simulink model "DF002A_Swp"  (R2013b)
settings: Solver=FixedStepDiscrete  StartTime=0  StopTime=350  FixedStep=ARCHGLBPRM_2MILLISEC_SEC_F32  RelTol=1e-3
undefined symbols (not defined in the file): ARCHGLBPRM_2MILLISEC_SEC_F32, ARCHGLBPRM_2PI_ULS_F32, SwpCfg, SwpDwellTi, SwpFrqList, SwpGain, SwpModEna, SwpOffs, SwpSinAmp, SWPTIUNITCNVN, SwpTranTi, SwpVehSpdChkEna, SwpVehSpdMax
libraries: simulink x6, NexteerUtilities x2
(part 2 of 2)

== system DF002A_Swp/Swp/DF002A Sweep Function/ SwpPer1/Check GenHwTrq and VehSpd/If GenHwTrq=TRUE, Check Vehicle Speed Criteria/Switch Case Block/Dwell//Stop: Switch Case Action Subsystem1/Cosine Calculation ==
  note: This constant defined as a
      | PIM in data dictionary
  note: This constant defined as a
      | PIM in data dictionary
  SinArg : Inport
  SF : Inport  Port=2
  Constant1 : Constant  Value=SwpSinAmp
  Constant3 : Constant  Value=SwpOffs
  Gain2 : Gain  Gain=ARCHGLBPRM_2PI_ULS_F32
  Product1 : Product  RndMeth=Zero
  Product2 : Product  RndMeth=Zero
  Sum4 : Sum  Inputs=|++
  Trigonometric Function : Trigonometry  Operator=cos
  Out1 : Outport
  wires:
  Gain2/1 -> Trigonometric Function/1
  Product2/1 -> Out1/1
  SinArg/1 -> Gain2/1
  Sum4/1 -> Product2/1
  Product1/1 -> Sum4/1
  Trigonometric Function/1 -> Product1/2
  SF/1 -> Product2/2
  Constant1/1 -> Product1/1  "SwpSinAmp"
  Constant3/1 -> Sum4/2  "SwpOffs"

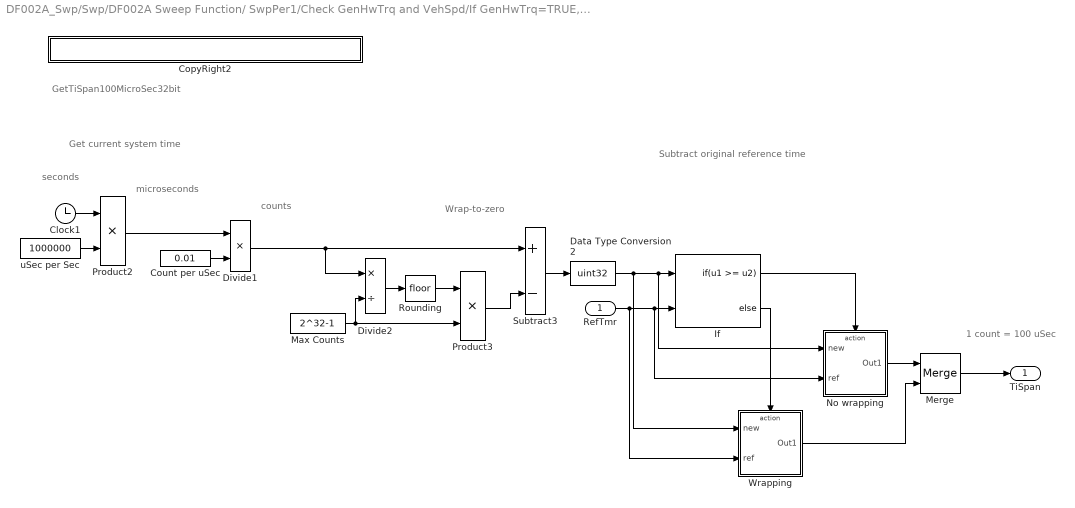
== system DF002A_Swp/Swp/DF002A Sweep Function/ SwpPer1/Check GenHwTrq and VehSpd/If GenHwTrq=TRUE, Check Vehicle Speed Criteria/Switch Case Block/Dwell//Stop: Switch Case Action Subsystem1/GetTiSpan100MicroSec32bit1 ==
  note: GetTiSpan100MicroSec32bit
  note: Get current system time
  note: 1 count = 100 uSec
  note: Wrap-to-zero
  note: counts
  note: microseconds
  note: seconds
  note: Subtract original reference time
  RefTmr : Inport
  Clock1 : Clock
  CopyRight2 : Subsystem  Description=|  mask(Copyright Information){none=on}
      | Copyright info block.                                               
      |                                                                     
      | Place copyright information at the top of every subsystem in design.
      mask prompts: none "No parameters"
      mask help: Place copyright information at the top of every subsystem in design.
      mask Display:
      | NxtrConf = 'Nexteer Confidential';
      | 
      | sys = bdroot; %handle for the current model ("system")
      | first = get_param(sys,'Created');
      | if(isempty(first))
      |     first = datestr(now,'yyyy');
      | else
      |     first = first(end-3:end);  %year is last four digits
      | end
      | 
      | last = get_param(sys,'LastModifiedDate');
      | if isempty(last)
      |     last = datestr(now,'yyyy');
      | else
      |     last = last(end-3:end);
      | end
      | 
      | if strcmp(first,last)
      |     fprintf('%s -- Copyright %s Nexteer',NxtrConf,first)
      | else
      |     fprintf('%s -- %s%s- %s Nexteer',NxtrConf,char(169),first,last)
      | end
  Count per uSec : Constant  Value=0.01
  Data Type Conversion2 : DataTypeConversion  OutDataTypeStr=uint32
  Divide1 : Product  Inputs=**
  Divide2 : Product  Inputs=*/
  If : If  NumInputs=2  IfExpression=u1 >= u2
  Max Counts : Constant  Value=2^32-1
  Merge : Merge
  No wrapping : Subsystem  TreatAsAtomicUnit=on
  Product2 : Product
  Product3 : Product
  Rounding : Rounding
  Subtract3 : Sum  Inputs=+-
  Wrapping : Subsystem  TreatAsAtomicUnit=on
  uSec per Sec : Constant  Value=1000000
  TiSpan : Outport
  wires:
  Data Type Conversion2/1 -> Wrapping/1(new), No wrapping/1(new), If/1
  RefTmr/1 -> Wrapping/2(ref), No wrapping/2(ref), If/2
  Merge/1 -> TiSpan/1
  uSec per Sec/1 -> Product2/2
  Count per uSec/1 -> Divide1/2
  Clock1/1 -> Product2/1
  Product2/1 -> Divide1/1
  Divide1/1 -> Subtract3/1, Divide2/1
  Max Counts/1 -> Product3/2, Divide2/2
  Divide2/1 -> Rounding/1
  Rounding/1 -> Product3/1
  Subtract3/1 -> Data Type Conversion2/1
  Product3/1 -> Subtract3/2
  If/1 -> No wrapping/Action
  If/2 -> Wrapping/Action
  No wrapping/1(Out1) -> Merge/1
  Wrapping/1(Out1) -> Merge/2

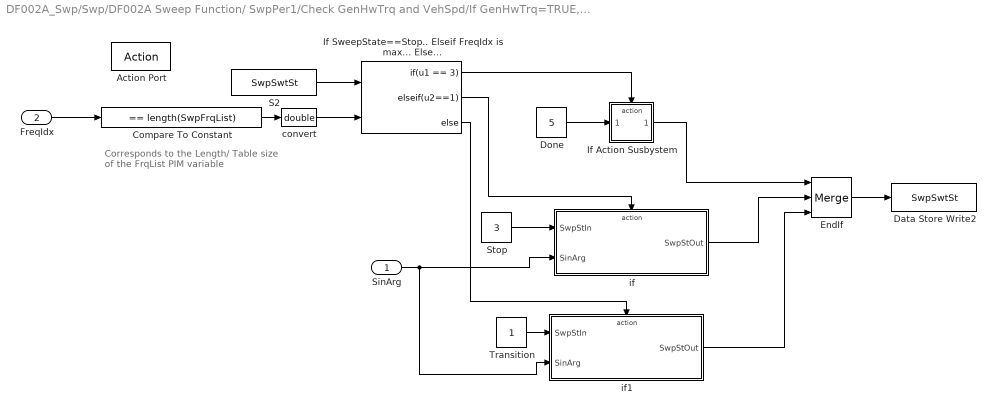
== system DF002A_Swp/Swp/DF002A Sweep Function/ SwpPer1/Check GenHwTrq and VehSpd/If GenHwTrq=TRUE, Check Vehicle Speed Criteria/Switch Case Block/Dwell//Stop: Switch Case Action Subsystem1/If Action Subsystem ==
  note: Corresponds to the Length/ Table size
      | of the FrqList  PIM variable
  SinArg : Inport
  FreqIdx : Inport  Port=2
  Action Port : ActionPort  ActionType=then
  Compare To Constant : simulink/Logic and Bit Operations/Compare To Constant  relop===  const=length(SwpFrqList)  OutDataTypeStr=boolean
      settings: AttributesFormatString=%<const>
  Data Store Write2 : DataStoreWrite  RequirementInfo={} %GIDa_98c06136_1203_45eb_bd39_84f10c760bb6  DataStoreName=SwpSwtSt
  Done : Constant  Value=5
  EndIf : Merge  Inputs=3
  If Action Susbystem : Subsystem  TreatAsAtomicUnit=on  mask(pass thru, version Nov 30, 2012){nIn=1}
      mask prompts: nIn "Number of input signals"
      mask help:
      | This block passes its input straight through without modification.
      |
      | Enter the number of signals to pass through (integer 1 to 5).
      mask Callback nIn:
      | thisBlock = gcb;
      | a = get_param(thisBlock,'MaskValues');
      | b = cell2mat(a);
      | c = str2num(b);
      | 
      | if c<1 c=1; end
      | if c>5 c=5; end
      | 
      | for idx=1:c
      |     sIdx = num2str(idx);
      |     oldblock = [thisBlock '/In' sIdx];
      |     if strcmp(get_param(oldblock,'BlockType'),'Ground')
      |          newblock = 'built-in/Inport';
      |         pos = get_param(oldblock,'Position');
      |         orient = get_param(oldblock,'Orientation');
      |         delete_block(oldblock);
      |         add_block(newblock,oldblock,'Position',pos, 'Orientation',orient);
      |     end
      | 
      |     oldblock = [thisBlock '/Out' sIdx];
      |     if strcmp(get_param(oldblock,'BlockType'),'Terminator')
      |         newblock = 'built-in/Outport';
      |         pos = get_param(oldblock,'Position');
      |         orient = get_param(oldblock,'Orientation');
      |         delete_block(oldblock);
      |         add_block(newblock,oldblock,'Position',pos, 'Orientation',orient);
      |     end
      | end
      | 
      | for idx=c+1:5
      |     sIdx = num2str(idx);
      |     oldblock = [thisBlock '/In' sIdx];
      |     if strcmp(get_param(oldblock,'BlockType'),'Inport')
      |         newblock = 'built-in/Ground';
      |         pos = get_param(oldblock,'Position');
      |         orient = get_param(oldblock,'Orientation');
      |         delete_block(oldblock);
      |         add_block(newblock,oldblock,'Position',pos, 'Orientation',orient);
      |     end
      | 
      |     oldblock = [thisBlock '/Out' sIdx];
      |     if strcmp(get_param(oldblock,'BlockType'),'Outport')
      |         newblock = 'built-in/Terminator';
      |         pos = get_param(oldblock,'Position');
      |         orient = get_param(oldblock,'Orientation');
      |         delete_block(oldblock);
      |         add_block(newblock,oldblock,'Position',pos, 'Orientation',orient);
      |     end
      | end
      | 
      | 
      | 
      | clear thisBlock oldblock newblock orient pos a b c idx sIdx ;
      mask Display: fprintf('pass\nthru')
  If SweepState==Stop.. Elseif FreqIdx is max... Else... : If  NumInputs=2  IfExpression=u1 == 3  ElseIfExpressions=u2==1
  S2 : DataStoreRead  DataStoreName=SwpSwtSt
  Stop : Constant  Value=3
  Transition : Constant
  convert : DataTypeConversion  OutDataTypeStr=double
  if : Subsystem  RequirementInfo={} %GIDa_0dc71279_9bfd_4c7e_903f_84cae79553a4  TreatAsAtomicUnit=on
  if1 : Subsystem  RequirementInfo={} %GIDa_9f322384_3993_4c4c_ad2a_ea70a5303c05  TreatAsAtomicUnit=on
  wires:
  S2/1 -> If SweepState==Stop.. Elseif FreqIdx is max... Else.../1
  If Action Susbystem/1(Out1) -> EndIf/1
  EndIf/1 -> Data Store Write2/1
  Done/1 -> If Action Susbystem/1(In1)
  If SweepState==Stop.. Elseif FreqIdx is max... Else.../1 -> If Action Susbystem/Action
  If SweepState==Stop.. Elseif FreqIdx is max... Else.../2 -> if/Action
  If SweepState==Stop.. Elseif FreqIdx is max... Else.../3 -> if1/Action
  FreqIdx/1 -> Compare To Constant/1
  Compare To Constant/1 -> convert/1
  convert/1 -> If SweepState==Stop.. Elseif FreqIdx is max... Else.../2
  Stop/1 -> if/1(SwpStIn)
  Transition/1 -> if1/1(SwpStIn)
  if/1(SwpStOut) -> EndIf/2
  if1/1(SwpStOut) -> EndIf/3
  SinArg/1 -> if1/2(SinArg), if/2(SinArg)

== system DF002A_Swp/Swp/DF002A Sweep Function/ SwpPer1/Check GenHwTrq and VehSpd/If GenHwTrq=TRUE, Check Vehicle Speed Criteria/Switch Case Block/Dwell//Stop: Switch Case Action Subsystem1/If Action Subsystem1 ==
  TransitionTime : Inport
  TimeScale : Inport  Port=2
  Action Port : ActionPort  ActionType=then
  Constant1 : Constant
  Sum : Sum  Inputs=|-+
  ScaleFactor : Outport
  StateTime : Outport  Port=2
  wires:
  TimeScale/1 -> Sum/1  "TimeScale_Uls_T_f32"
  Constant1/1 -> Sum/2
  TransitionTime/1 -> StateTime/1
  Sum/1 -> ScaleFactor/1

== system DF002A_Swp/Swp/DF002A Sweep Function/ SwpPer1/Check GenHwTrq and VehSpd/If GenHwTrq=TRUE, Check Vehicle Speed Criteria/Switch Case Block/Dwell//Stop: Switch Case Action Subsystem1/If Action Subsystem2 ==
  DwellTime : Inport
  Action Port : ActionPort  ActionType=else
  Constant2 : Constant
  ScaleFactor : Outport
  StateTime : Outport  Port=2
  wires:
  DwellTime/1 -> StateTime/1
  Constant2/1 -> ScaleFactor/1

== system DF002A_Swp/Swp/DF002A Sweep Function/ SwpPer1/Check GenHwTrq and VehSpd/If GenHwTrq=TRUE, Check Vehicle Speed Criteria/Switch Case Block/Dwell//Stop: Switch Case Action Subsystem1/Inst Frequency Calculation ==
  note: This block find instantaneous frequency of the sinusoid signal during dwell/stop case.
      | Since the frequency is held constand during either of these cases, InstFreq=CurrentFreq
  CurrentFreq : Inport
  InstFreq : Outport
  wires:
  CurrentFreq/1 -> InstFreq/1

== system DF002A_Swp/Swp/DF002A Sweep Function/ SwpPer1/Check GenHwTrq and VehSpd/If GenHwTrq=TRUE, Check Vehicle Speed Criteria/Switch Case Block/Dwell//Stop: Switch Case Action Subsystem1/Sine Calculation ==
  note: This constant defined as a
      | PIM in data dictionary
  note: This constant defined as a
      | PIM in data dictionary
  SinArg : Inport
  SF : Inport  Port=2
  Constant3 : Constant  Value=SwpOffs
  Constant4 : Constant  Value=SwpSinAmp
  Gain2 : Gain  Gain=ARCHGLBPRM_2PI_ULS_F32
  Product1 : Product  RndMeth=Zero
  Product2 : Product  RndMeth=Zero
  Sum4 : Sum  Inputs=|++
  Trigonometric Function : Trigonometry
  Out1 : Outport
  wires:
  Gain2/1 -> Trigonometric Function/1
  Product2/1 -> Out1/1
  SinArg/1 -> Gain2/1
  Sum4/1 -> Product2/1
  Product1/1 -> Sum4/1
  Constant4/1 -> Product1/1  "SwpSinAmp"
  Trigonometric Function/1 -> Product1/2
  SF/1 -> Product2/2
  Constant3/1 -> Sum4/2  "SwpOffs"

== system DF002A_Swp/Swp/DF002A Sweep Function/ SwpPer1/Check GenHwTrq and VehSpd/If GenHwTrq=TRUE, Check Vehicle Speed Criteria/Switch Case Block/Ramp: Switch Case Action/Else Action Subsystem ==
  SweepTorqueIn : Inport
  CosSweepTorqueIn : Inport  Port=2
  ScaleFactor : Inport  Port=3
  Action Port : ActionPort  ActionType=else
  Product : Product  RndMeth=Zero
  Product1 : Product  RndMeth=Zero
  SweepTorque : Outport
  CosSweepTorque : Outport  Port=2
  wires:
  CosSweepTorqueIn/1 -> Product1/2
  ScaleFactor/1 -> Product/2, Product1/1
  Product/1 -> SweepTorque/1
  Product1/1 -> CosSweepTorque/1
  SweepTorqueIn/1 -> Product/1

== system DF002A_Swp/Swp/DF002A Sweep Function/ SwpPer1/Check GenHwTrq and VehSpd/If GenHwTrq=TRUE, Check Vehicle Speed Criteria/Switch Case Block/Ramp: Switch Case Action/Else Action Subsystem1 ==
  Action Port : ActionPort  ActionType=then
  Constant : Constant  Value=0
  Constant1 : Constant  Value=0
  Data Store Write2 : DataStoreWrite  RequirementInfo={} %GIDa_95120470_507b_4450_bc77_8b8934b75d51  DataStoreName=SwpSwtSt
  DefaultSweepState (DONE) : Constant  Value=5
  SweepTorque : Outport
  CosSweepTorque : Outport  Port=2
  wires:
  Constant/1 -> SweepTorque/1
  Constant1/1 -> CosSweepTorque/1
  DefaultSweepState (DONE)/1 -> Data Store Write2/1

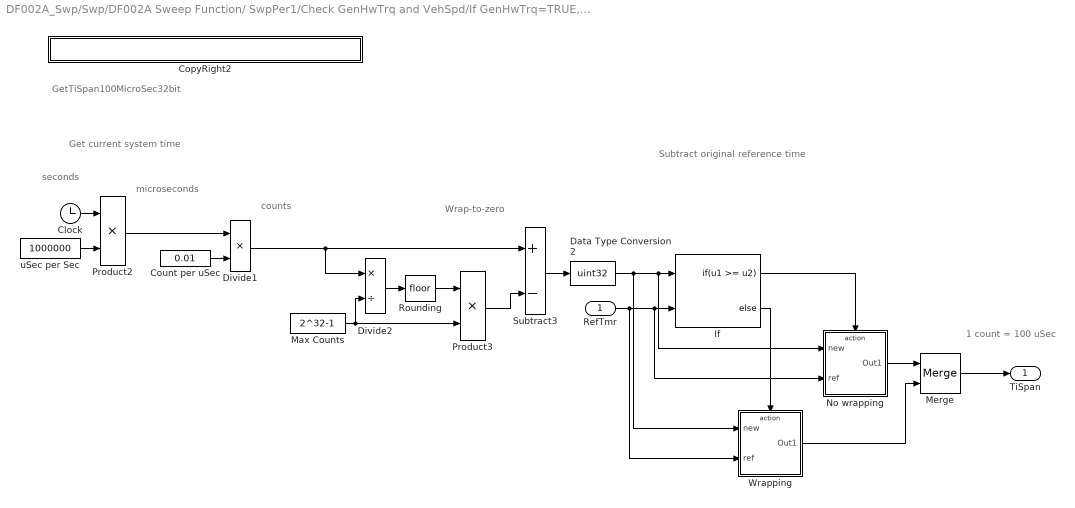
== system DF002A_Swp/Swp/DF002A Sweep Function/ SwpPer1/Check GenHwTrq and VehSpd/If GenHwTrq=TRUE, Check Vehicle Speed Criteria/Switch Case Block/Ramp: Switch Case Action/GetTiSpan100MicroSec32bit1 ==
  note: GetTiSpan100MicroSec32bit
  note: Get current system time
  note: 1 count = 100 uSec
  note: Wrap-to-zero
  note: counts
  note: microseconds
  note: seconds
  note: Subtract original reference time
  RefTmr : Inport
  Clock : Clock
  CopyRight2 : Subsystem  Description=|  mask(Copyright Information){none=on}
      | Copyright info block.                                               
      |                                                                     
      | Place copyright information at the top of every subsystem in design.
      mask prompts: none "No parameters"
      mask help: Place copyright information at the top of every subsystem in design.
      mask Display:
      | NxtrConf = 'Nexteer Confidential';
      | 
      | sys = bdroot; %handle for the current model ("system")
      | first = get_param(sys,'Created');
      | if(isempty(first))
      |     first = datestr(now,'yyyy');
      | else
      |     first = first(end-3:end);  %year is last four digits
      | end
      | 
      | last = get_param(sys,'LastModifiedDate');
      | if isempty(last)
      |     last = datestr(now,'yyyy');
      | else
      |     last = last(end-3:end);
      | end
      | 
      | if strcmp(first,last)
      |     fprintf('%s -- Copyright %s Nexteer',NxtrConf,first)
      | else
      |     fprintf('%s -- %s%s- %s Nexteer',NxtrConf,char(169),first,last)
      | end
  Count per uSec : Constant  Value=0.01
  Data Type Conversion2 : DataTypeConversion  OutDataTypeStr=uint32
  Divide1 : Product  Inputs=**
  Divide2 : Product  Inputs=*/
  If : If  NumInputs=2  IfExpression=u1 >= u2
  Max Counts : Constant  Value=2^32-1
  Merge : Merge
  No wrapping : Subsystem  TreatAsAtomicUnit=on
  Product2 : Product
  Product3 : Product
  Rounding : Rounding
  Subtract3 : Sum  Inputs=+-
  Wrapping : Subsystem  TreatAsAtomicUnit=on
  uSec per Sec : Constant  Value=1000000
  TiSpan : Outport
  wires:
  Data Type Conversion2/1 -> Wrapping/1(new), No wrapping/1(new), If/1
  RefTmr/1 -> Wrapping/2(ref), No wrapping/2(ref), If/2
  Merge/1 -> TiSpan/1
  uSec per Sec/1 -> Product2/2
  Count per uSec/1 -> Divide1/2
  Clock/1 -> Product2/1
  Product2/1 -> Divide1/1
  Divide1/1 -> Subtract3/1, Divide2/1
  Max Counts/1 -> Product3/2, Divide2/2
  Divide2/1 -> Rounding/1
  Rounding/1 -> Product3/1
  Subtract3/1 -> Data Type Conversion2/1
  Product3/1 -> Subtract3/2
  If/1 -> No wrapping/Action
  If/2 -> Wrapping/Action
  No wrapping/1(Out1) -> Merge/1
  Wrapping/1(Out1) -> Merge/2

== system DF002A_Swp/Swp/DF002A Sweep Function/ SwpPer1/Check GenHwTrq and VehSpd/If GenHwTrq=TRUE, Check Vehicle Speed Criteria/Switch Case Block/Start//Transition: Switch Case Action Subsystem /Cosine Calculation ==
  note: This constant defined as a
      | PIM in data dictionary
  note: This constant defined as a
      | PIM in data dictionary
  SF : Inport
  SinArg : Inport  Port=2
  Constant3 : Constant  Value=SwpOffs
  Constant4 : Constant  Value=SwpSinAmp
  Gain2 : Gain  Gain=ARCHGLBPRM_2PI_ULS_F32
  Product1 : Product  RndMeth=Zero
  Product2 : Product  RndMeth=Zero
  Sum4 : Sum  Inputs=|++
  Trigonometric Function : Trigonometry  Operator=cos
  Out1 : Outport
  wires:
  Gain2/1 -> Trigonometric Function/1
  Product2/1 -> Out1/1
  SinArg/1 -> Gain2/1
  Sum4/1 -> Product2/1
  Product1/1 -> Sum4/1
  Trigonometric Function/1 -> Product1/2
  Constant3/1 -> Sum4/2  "SwpOffs"
  SF/1 -> Product2/2
  Constant4/1 -> Product1/1  "SwpSinAmp"

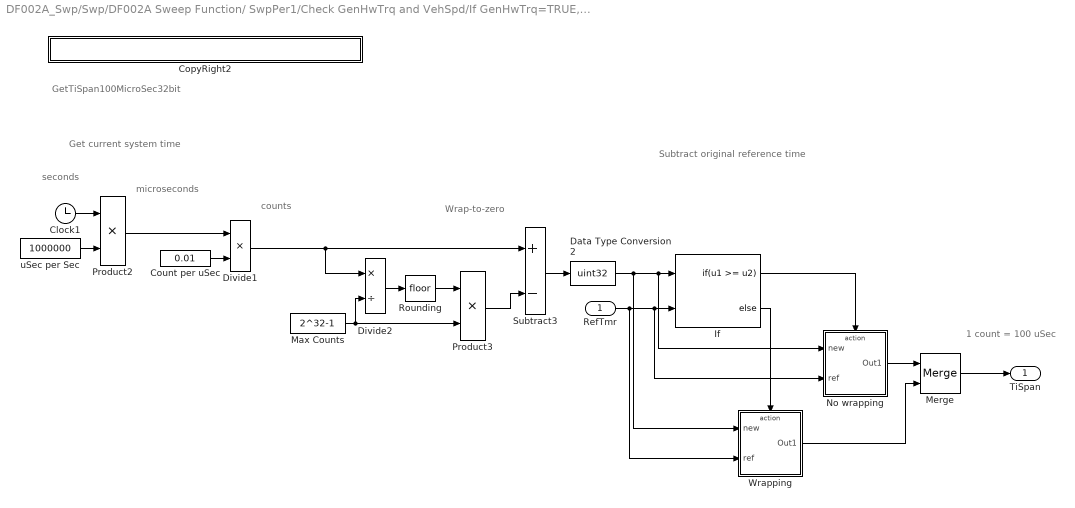
== system DF002A_Swp/Swp/DF002A Sweep Function/ SwpPer1/Check GenHwTrq and VehSpd/If GenHwTrq=TRUE, Check Vehicle Speed Criteria/Switch Case Block/Start//Transition: Switch Case Action Subsystem /GetTiSpan100MicroSec32bit1 ==
  note: GetTiSpan100MicroSec32bit
  note: Get current system time
  note: 1 count = 100 uSec
  note: Wrap-to-zero
  note: counts
  note: microseconds
  note: seconds
  note: Subtract original reference time
  RefTmr : Inport
  Clock1 : Clock
  CopyRight2 : Subsystem  Description=|  mask(Copyright Information){none=on}
      | Copyright info block.                                               
      |                                                                     
      | Place copyright information at the top of every subsystem in design.
      mask prompts: none "No parameters"
      mask help: Place copyright information at the top of every subsystem in design.
      mask Display:
      | NxtrConf = 'Nexteer Confidential';
      | 
      | sys = bdroot; %handle for the current model ("system")
      | first = get_param(sys,'Created');
      | if(isempty(first))
      |     first = datestr(now,'yyyy');
      | else
      |     first = first(end-3:end);  %year is last four digits
      | end
      | 
      | last = get_param(sys,'LastModifiedDate');
      | if isempty(last)
      |     last = datestr(now,'yyyy');
      | else
      |     last = last(end-3:end);
      | end
      | 
      | if strcmp(first,last)
      |     fprintf('%s -- Copyright %s Nexteer',NxtrConf,first)
      | else
      |     fprintf('%s -- %s%s- %s Nexteer',NxtrConf,char(169),first,last)
      | end
  Count per uSec : Constant  Value=0.01
  Data Type Conversion2 : DataTypeConversion  OutDataTypeStr=uint32
  Divide1 : Product  Inputs=**
  Divide2 : Product  Inputs=*/
  If : If  NumInputs=2  IfExpression=u1 >= u2
  Max Counts : Constant  Value=2^32-1
  Merge : Merge
  No wrapping : Subsystem  TreatAsAtomicUnit=on
  Product2 : Product
  Product3 : Product
  Rounding : Rounding
  Subtract3 : Sum  Inputs=+-
  Wrapping : Subsystem  TreatAsAtomicUnit=on
  uSec per Sec : Constant  Value=1000000
  TiSpan : Outport
  wires:
  Data Type Conversion2/1 -> Wrapping/1(new), No wrapping/1(new), If/1
  RefTmr/1 -> Wrapping/2(ref), No wrapping/2(ref), If/2
  Merge/1 -> TiSpan/1
  uSec per Sec/1 -> Product2/2
  Count per uSec/1 -> Divide1/2
  Clock1/1 -> Product2/1
  Product2/1 -> Divide1/1
  Divide1/1 -> Subtract3/1, Divide2/1
  Max Counts/1 -> Product3/2, Divide2/2
  Divide2/1 -> Rounding/1
  Rounding/1 -> Product3/1
  Subtract3/1 -> Data Type Conversion2/1
  Product3/1 -> Subtract3/2
  If/1 -> No wrapping/Action
  If/2 -> Wrapping/Action
  No wrapping/1(Out1) -> Merge/1
  Wrapping/1(Out1) -> Merge/2

== system DF002A_Swp/Swp/DF002A Sweep Function/ SwpPer1/Check GenHwTrq and VehSpd/If GenHwTrq=TRUE, Check Vehicle Speed Criteria/Switch Case Block/Start//Transition: Switch Case Action Subsystem /Inst Frequency Calculation ==
  note: This block find instantaneous frequency of the sinusoid signal during start/transition case.
  TimeScale : Inport
  InitialFreq : Inport  Port=2
  FreqSpan : Inport  Port=3
  Product1 : Product  RndMeth=Zero
  Sum4 : Sum
  InstFreq : Outport
  wires:
  FreqSpan/1 -> Product1/1
  Sum4/1 -> InstFreq/1
  TimeScale/1 -> Product1/2
  Product1/1 -> Sum4/1  "DeltaFreq"
  InitialFreq/1 -> Sum4/2

== system DF002A_Swp/Swp/DF002A Sweep Function/ SwpPer1/Check GenHwTrq and VehSpd/If GenHwTrq=TRUE, Check Vehicle Speed Criteria/Switch Case Block/Start//Transition: Switch Case Action Subsystem /ScaleFactor Calculation ==
  note: Note: FreqIdx starts with 1 in MATLAB. For C code one may have to use 0 as starting index.
  TimeScale : Inport
  FreqIdx : Inport  Port=2
  Constant1 : Constant
  If : If  IfExpression=u1 == 1
  If Action Subsystem : Subsystem  TreatAsAtomicUnit=on  mask(pass thru, version Nov 30, 2012){nIn=1}
      mask prompts: nIn "Number of input signals"
      mask help:
      | This block passes its input straight through without modification.
      |
      | Enter the number of signals to pass through (integer 1 to 5).
      mask Callback nIn:
      | thisBlock = gcb;
      | a = get_param(thisBlock,'MaskValues');
      | b = cell2mat(a);
      | c = str2num(b);
      | 
      | if c<1 c=1; end
      | if c>5 c=5; end
      | 
      | for idx=1:c
      |     sIdx = num2str(idx);
      |     oldblock = [thisBlock '/In' sIdx];
      |     if strcmp(get_param(oldblock,'BlockType'),'Ground')
      |          newblock = 'built-in/Inport';
      |         pos = get_param(oldblock,'Position');
      |         orient = get_param(oldblock,'Orientation');
      |         delete_block(oldblock);
      |         add_block(newblock,oldblock,'Position',pos, 'Orientation',orient);
      |     end
      | 
      |     oldblock = [thisBlock '/Out' sIdx];
      |     if strcmp(get_param(oldblock,'BlockType'),'Terminator')
      |         newblock = 'built-in/Outport';
      |         pos = get_param(oldblock,'Position');
      |         orient = get_param(oldblock,'Orientation');
      |         delete_block(oldblock);
      |         add_block(newblock,oldblock,'Position',pos, 'Orientation',orient);
      |     end
      | end
      | 
      | for idx=c+1:5
      |     sIdx = num2str(idx);
      |     oldblock = [thisBlock '/In' sIdx];
      |     if strcmp(get_param(oldblock,'BlockType'),'Inport')
      |         newblock = 'built-in/Ground';
      |         pos = get_param(oldblock,'Position');
      |         orient = get_param(oldblock,'Orientation');
      |         delete_block(oldblock);
      |         add_block(newblock,oldblock,'Position',pos, 'Orientation',orient);
      |     end
      | 
      |     oldblock = [thisBlock '/Out' sIdx];
      |     if strcmp(get_param(oldblock,'BlockType'),'Outport')
      |         newblock = 'built-in/Terminator';
      |         pos = get_param(oldblock,'Position');
      |         orient = get_param(oldblock,'Orientation');
      |         delete_block(oldblock);
      |         add_block(newblock,oldblock,'Position',pos, 'Orientation',orient);
      |     end
      | end
      | 
      | 
      | 
      | clear thisBlock oldblock newblock orient pos a b c idx sIdx ;
      mask Display: fprintf('pass\nthru')
  ScaleFactorMerge : Merge
  Then Action Subsystem : Subsystem  TreatAsAtomicUnit=on  mask(pass thru, version Nov 30, 2012){nIn=1}
      mask prompts: nIn "Number of input signals"
      mask help:
      | This block passes its input straight through without modification.
      |
      | Enter the number of signals to pass through (integer 1 to 5).
      mask Callback nIn:
      | thisBlock = gcb;
      | a = get_param(thisBlock,'MaskValues');
      | b = cell2mat(a);
      | c = str2num(b);
      | 
      | if c<1 c=1; end
      | if c>5 c=5; end
      | 
      | for idx=1:c
      |     sIdx = num2str(idx);
      |     oldblock = [thisBlock '/In' sIdx];
      |     if strcmp(get_param(oldblock,'BlockType'),'Ground')
      |          newblock = 'built-in/Inport';
      |         pos = get_param(oldblock,'Position');
      |         orient = get_param(oldblock,'Orientation');
      |         delete_block(oldblock);
      |         add_block(newblock,oldblock,'Position',pos, 'Orientation',orient);
      |     end
      | 
      |     oldblock = [thisBlock '/Out' sIdx];
      |     if strcmp(get_param(oldblock,'BlockType'),'Terminator')
      |         newblock = 'built-in/Outport';
      |         pos = get_param(oldblock,'Position');
      |         orient = get_param(oldblock,'Orientation');
      |         delete_block(oldblock);
      |         add_block(newblock,oldblock,'Position',pos, 'Orientation',orient);
      |     end
      | end
      | 
      | for idx=c+1:5
      |     sIdx = num2str(idx);
      |     oldblock = [thisBlock '/In' sIdx];
      |     if strcmp(get_param(oldblock,'BlockType'),'Inport')
      |         newblock = 'built-in/Ground';
      |         pos = get_param(oldblock,'Position');
      |         orient = get_param(oldblock,'Orientation');
      |         delete_block(oldblock);
      |         add_block(newblock,oldblock,'Position',pos, 'Orientation',orient);
      |     end
      | 
      |     oldblock = [thisBlock '/Out' sIdx];
      |     if strcmp(get_param(oldblock,'BlockType'),'Outport')
      |         newblock = 'built-in/Terminator';
      |         pos = get_param(oldblock,'Position');
      |         orient = get_param(oldblock,'Orientation');
      |         delete_block(oldblock);
      |         add_block(newblock,oldblock,'Position',pos, 'Orientation',orient);
      |     end
      | end
      | 
      | 
      | 
      | clear thisBlock oldblock newblock orient pos a b c idx sIdx ;
      mask Display: fprintf('pass\nthru')
  ScaleFactor : Outport
  wires:
  If/2 -> Then Action Subsystem/Action
  Constant1/1 -> Then Action Subsystem/1(In1)
  If Action Subsystem/1(Out1) -> ScaleFactorMerge/1
  Then Action Subsystem/1(Out1) -> ScaleFactorMerge/2
  TimeScale/1 -> If Action Subsystem/1(In1)
  FreqIdx/1 -> If/1
  ScaleFactorMerge/1 -> ScaleFactor/1
  If/1 -> If Action Subsystem/Action

== system DF002A_Swp/Swp/DF002A Sweep Function/ SwpPer1/Check GenHwTrq and VehSpd/If GenHwTrq=TRUE, Check Vehicle Speed Criteria/Switch Case Block/Start//Transition: Switch Case Action Subsystem /Sine Calculation ==
  note: This constant defined as a
      | PIM in data dictionary
  note: This constant defined as a
      | PIM in data dictionary
  SinArg : Inport
  SF : Inport  Port=2
  Constant3 : Constant  Value=SwpOffs
  Constant4 : Constant  Value=SwpSinAmp
  Gain2 : Gain  Gain=ARCHGLBPRM_2PI_ULS_F32
  Product1 : Product  RndMeth=Zero
  Product2 : Product  RndMeth=Zero
  Sum4 : Sum
  Trigonometric Function : Trigonometry
  Out1 : Outport
  wires:
  Gain2/1 -> Trigonometric Function/1
  Product2/1 -> Out1/1
  SinArg/1 -> Gain2/1
  Sum4/1 -> Product2/1
  Product1/1 -> Sum4/1
  Trigonometric Function/1 -> Product1/2
  SF/1 -> Product2/2
  Constant4/1 -> Product1/1  "SwpSinAmp"
  Constant3/1 -> Sum4/2  "SwpOffs"

== system DF002A_Swp/Swp/DF002A Sweep Function/ SwpPer1/Check GenHwTrq and VehSpd/If GenHwTrq=TRUE, Check Vehicle Speed Criteria/Switch Case Block/Start//Transition: Switch Case Action Subsystem /if ==
  SwpStIn : Inport
  SinArgIn : Inport  Port=2
  FreqIdx : Inport  Port=3
  Action Port : ActionPort  ActionType=then
  CopyRight2 : Subsystem  Description=|  mask(Copyright Information){none=on}
      | Copyright info block.                                               
      |                                                                     
      | Place copyright information at the top of every subsystem in design.
      mask prompts: none "No parameters"
      mask help: Place copyright information at the top of every subsystem in design.
      mask Display:
      | NxtrConf = 'Nexteer Confidential';
      | 
      | sys = bdroot; %handle for the current model ("system")
      | first = get_param(sys,'Created');
      | if(isempty(first))
      |     first = datestr(now,'yyyy');
      | else
      |     first = first(end-3:end);  %year is last four digits
      | end
      | 
      | last = get_param(sys,'LastModifiedDate');
      | if isempty(last)
      |     last = datestr(now,'yyyy');
      | else
      |     last = last(end-3:end);
      | end
      | 
      | if strcmp(first,last)
      |     fprintf('%s -- Copyright %s Nexteer',NxtrConf,first)
      | else
      |     fprintf('%s -- %s%s- %s Nexteer',NxtrConf,char(169),first,last)
      | end
  Data Store Write1 : DataStoreWrite  RequirementInfo={} %GIDa_2d5c68f4_9fd1_43d7_987e_96652c4ff694  DataStoreName=SwpDwellStrtTi
  Data Store Write2 : DataStoreWrite  RequirementInfo={} %GIDa_11008d3d_2985_4841_8276_11fe24cf555c  DataStoreName=SwpSwtSt
  Data Store Write3 : DataStoreWrite  RequirementInfo={} %GIDa_ff896d98_7f04_4da2_acbb_ed610564ff8c  DataStoreName=SwpLstStSinArg
  Data Store Write4 : DataStoreWrite  RequirementInfo={} %GIDa_120499b8_bbe6_4e64_beba_aa38302bffa2  DataStoreName=SwpFrqIdx
  GetRefTmr100MicroSec32bit : Subsystem  RequirementInfo={} %GIDa_e4c8ee1a_9b9e_4e76_8284_54106fdba1f2
  wires:
  GetRefTmr100MicroSec32bit/1(RefTmr) -> Data Store Write1/1
  SwpStIn/1 -> Data Store Write2/1
  SinArgIn/1 -> Data Store Write3/1
  FreqIdx/1 -> Data Store Write4/1

== system DF002A_Swp/Swp/DF002A Sweep Function/ SwpPer1/Check GenHwTrq and VehSpd/If GenHwTrq=TRUE, Check Vehicle Speed Criteria/if1/GetRefTmr100MicroSec32bit/CopyRight2 ==

== system DF002A_Swp/Swp/DF002A Sweep Function/ SwpPer1/Check GenHwTrq and VehSpd/If GenHwTrq=TRUE, Check Vehicle Speed Criteria/Switch Case Block/Dwell//Stop: Switch Case Action Subsystem1/GetTiSpan100MicroSec32bit1/CopyRight2 ==

== system DF002A_Swp/Swp/DF002A Sweep Function/ SwpPer1/Check GenHwTrq and VehSpd/If GenHwTrq=TRUE, Check Vehicle Speed Criteria/Switch Case Block/Dwell//Stop: Switch Case Action Subsystem1/GetTiSpan100MicroSec32bit1/No wrapping ==
  new : Inport
  ref : Inport  Port=2
  Action Port : ActionPort  ActionType=then
  Subtract1 : Sum  Inputs=+-
  Out1 : Outport
  wires:
  Subtract1/1 -> Out1/1
  new/1 -> Subtract1/1
  ref/1 -> Subtract1/2

== system DF002A_Swp/Swp/DF002A Sweep Function/ SwpPer1/Check GenHwTrq and VehSpd/If GenHwTrq=TRUE, Check Vehicle Speed Criteria/Switch Case Block/Dwell//Stop: Switch Case Action Subsystem1/GetTiSpan100MicroSec32bit1/Wrapping ==
  new : Inport
  ref : Inport  Port=2
  Action Port : ActionPort  ActionType=else
  Max Counts : Constant  Value=2^32-1  OutDataTypeStr=uint32
  Subtract1 : Sum  Inputs=+-+
  Out1 : Outport
  wires:
  Subtract1/1 -> Out1/1
  Max Counts/1 -> Subtract1/1
  ref/1 -> Subtract1/2
  new/1 -> Subtract1/3

== system DF002A_Swp/Swp/DF002A Sweep Function/ SwpPer1/Check GenHwTrq and VehSpd/If GenHwTrq=TRUE, Check Vehicle Speed Criteria/Switch Case Block/Dwell//Stop: Switch Case Action Subsystem1/If Action Subsystem/If Action Susbystem ==
  note: Change Log:
      | Oct 12, 2012  Created by Kevin Derry as a 1-input, 1-output block
      | Nov 30, 2012  dynamically configurable for 1 to 5 ports.
  note: Do not modify these blocks manually.  They
      | are generated programatically.  Changing the
      | number of blocks available or their names requires
      | corresponding changes to Callback and Initialization
      | routines.
      |
      | Do not change the "Display" tab of mask editor.  The
      | outport names are created programatically in the
      | "Initialize" section.
  In1 : Inport
  Action Port : ActionPort  ActionType=then
  In{2..5} (4 alike) : Ground
  Out{2..5} (4 alike) : Terminator
  Out1 : Outport
  wires:
  In1/1 -> Out1/1
  In2/1 -> Out2/1
  In3/1 -> Out3/1
  In4/1 -> Out4/1
  In5/1 -> Out5/1

== system DF002A_Swp/Swp/DF002A Sweep Function/ SwpPer1/Check GenHwTrq and VehSpd/If GenHwTrq=TRUE, Check Vehicle Speed Criteria/Switch Case Block/Dwell//Stop: Switch Case Action Subsystem1/If Action Subsystem/if ==
  SwpStIn : Inport
  SinArg : Inport  Port=2
  Action Port : ActionPort  ActionType=elseif
  CopyRight2 : Subsystem  Description=|  mask(Copyright Information){none=on}
      | Copyright info block.                                               
      |                                                                     
      | Place copyright information at the top of every subsystem in design.
      mask prompts: none "No parameters"
      mask help: Place copyright information at the top of every subsystem in design.
      mask Display:
      | NxtrConf = 'Nexteer Confidential';
      | 
      | sys = bdroot; %handle for the current model ("system")
      | first = get_param(sys,'Created');
      | if(isempty(first))
      |     first = datestr(now,'yyyy');
      | else
      |     first = first(end-3:end);  %year is last four digits
      | end
      | 
      | last = get_param(sys,'LastModifiedDate');
      | if isempty(last)
      |     last = datestr(now,'yyyy');
      | else
      |     last = last(end-3:end);
      | end
      | 
      | if strcmp(first,last)
      |     fprintf('%s -- Copyright %s Nexteer',NxtrConf,first)
      | else
      |     fprintf('%s -- %s%s- %s Nexteer',NxtrConf,char(169),first,last)
      | end
  Data Store Write1 : DataStoreWrite  RequirementInfo={} %GIDa_4f1e3d04_d9e7_4733_8fd8_262fd0a3eb8f  DataStoreName=SwpDwellStrtTi
  Data Store Write2 : DataStoreWrite  RequirementInfo={} %GIDa_d48ca7cb_61a6_42aa_a34b_5bf9b1296ece  DataStoreName=SwpLstStSinArg
  GetRefTmr100MicroSec32bit : Subsystem  RequirementInfo={} %GIDa_68ed5a90_26e2_41ad_ad39_f0c5ffdf3187
  SwpStOut : Outport
  wires:
  GetRefTmr100MicroSec32bit/1(RefTmr) -> Data Store Write1/1
  SwpStIn/1 -> SwpStOut/1
  SinArg/1 -> Data Store Write2/1

== system DF002A_Swp/Swp/DF002A Sweep Function/ SwpPer1/Check GenHwTrq and VehSpd/If GenHwTrq=TRUE, Check Vehicle Speed Criteria/Switch Case Block/Dwell//Stop: Switch Case Action Subsystem1/If Action Subsystem/if1 ==
  SwpStIn : Inport
  SinArg : Inport  Port=2
  Action Port : ActionPort  ActionType=else
  CopyRight2 : Subsystem  Description=|  mask(Copyright Information){none=on}
      | Copyright info block.                                               
      |                                                                     
      | Place copyright information at the top of every subsystem in design.
      mask prompts: none "No parameters"
      mask help: Place copyright information at the top of every subsystem in design.
      mask Display:
      | NxtrConf = 'Nexteer Confidential';
      | 
      | sys = bdroot; %handle for the current model ("system")
      | first = get_param(sys,'Created');
      | if(isempty(first))
      |     first = datestr(now,'yyyy');
      | else
      |     first = first(end-3:end);  %year is last four digits
      | end
      | 
      | last = get_param(sys,'LastModifiedDate');
      | if isempty(last)
      |     last = datestr(now,'yyyy');
      | else
      |     last = last(end-3:end);
      | end
      | 
      | if strcmp(first,last)
      |     fprintf('%s -- Copyright %s Nexteer',NxtrConf,first)
      | else
      |     fprintf('%s -- %s%s- %s Nexteer',NxtrConf,char(169),first,last)
      | end
  Data Store Write1 : DataStoreWrite  RequirementInfo={} %GIDa_f83dc640_bc0b_49ad_a3ef_cfcad0b2b407  DataStoreName=SwpTranStrtTi
  Data Store Write2 : DataStoreWrite  RequirementInfo={} %GIDa_d830fb78_baaf_4cc4_8cbd_a7696e693b6b  DataStoreName=SwpLstStSinArg
  GetRefTmr100MicroSec32bit : Subsystem  RequirementInfo={} %GIDa_43d9dc88_264b_45e1_a75e_5b1b4b23420f
  SwpStOut : Outport
  wires:
  GetRefTmr100MicroSec32bit/1(RefTmr) -> Data Store Write1/1
  SwpStIn/1 -> SwpStOut/1
  SinArg/1 -> Data Store Write2/1

== system DF002A_Swp/Swp/DF002A Sweep Function/ SwpPer1/Check GenHwTrq and VehSpd/If GenHwTrq=TRUE, Check Vehicle Speed Criteria/Switch Case Block/Ramp: Switch Case Action/GetTiSpan100MicroSec32bit1/CopyRight2 ==

== system DF002A_Swp/Swp/DF002A Sweep Function/ SwpPer1/Check GenHwTrq and VehSpd/If GenHwTrq=TRUE, Check Vehicle Speed Criteria/Switch Case Block/Ramp: Switch Case Action/GetTiSpan100MicroSec32bit1/No wrapping ==
  new : Inport
  ref : Inport  Port=2
  Action Port : ActionPort  ActionType=then
  Subtract1 : Sum  Inputs=+-
  Out1 : Outport
  wires:
  Subtract1/1 -> Out1/1
  new/1 -> Subtract1/1
  ref/1 -> Subtract1/2

== system DF002A_Swp/Swp/DF002A Sweep Function/ SwpPer1/Check GenHwTrq and VehSpd/If GenHwTrq=TRUE, Check Vehicle Speed Criteria/Switch Case Block/Ramp: Switch Case Action/GetTiSpan100MicroSec32bit1/Wrapping ==
  new : Inport
  ref : Inport  Port=2
  Action Port : ActionPort  ActionType=else
  Max Counts : Constant  Value=2^32-1  OutDataTypeStr=uint32
  Subtract1 : Sum  Inputs=+-+
  Out1 : Outport
  wires:
  Subtract1/1 -> Out1/1
  Max Counts/1 -> Subtract1/1
  ref/1 -> Subtract1/2
  new/1 -> Subtract1/3

== system DF002A_Swp/Swp/DF002A Sweep Function/ SwpPer1/Check GenHwTrq and VehSpd/If GenHwTrq=TRUE, Check Vehicle Speed Criteria/Switch Case Block/Start//Transition: Switch Case Action Subsystem /GetTiSpan100MicroSec32bit1/CopyRight2 ==

== system DF002A_Swp/Swp/DF002A Sweep Function/ SwpPer1/Check GenHwTrq and VehSpd/If GenHwTrq=TRUE, Check Vehicle Speed Criteria/Switch Case Block/Start//Transition: Switch Case Action Subsystem /GetTiSpan100MicroSec32bit1/No wrapping ==
  new : Inport
  ref : Inport  Port=2
  Action Port : ActionPort  ActionType=then
  Subtract1 : Sum  Inputs=+-
  Out1 : Outport
  wires:
  Subtract1/1 -> Out1/1
  new/1 -> Subtract1/1
  ref/1 -> Subtract1/2

== system DF002A_Swp/Swp/DF002A Sweep Function/ SwpPer1/Check GenHwTrq and VehSpd/If GenHwTrq=TRUE, Check Vehicle Speed Criteria/Switch Case Block/Start//Transition: Switch Case Action Subsystem /GetTiSpan100MicroSec32bit1/Wrapping ==
  new : Inport
  ref : Inport  Port=2
  Action Port : ActionPort  ActionType=else
  Max Counts : Constant  Value=2^32-1  OutDataTypeStr=uint32
  Subtract1 : Sum  Inputs=+-+
  Out1 : Outport
  wires:
  Subtract1/1 -> Out1/1
  Max Counts/1 -> Subtract1/1
  ref/1 -> Subtract1/2
  new/1 -> Subtract1/3

== system DF002A_Swp/Swp/DF002A Sweep Function/ SwpPer1/Check GenHwTrq and VehSpd/If GenHwTrq=TRUE, Check Vehicle Speed Criteria/Switch Case Block/Start//Transition: Switch Case Action Subsystem /ScaleFactor Calculation/If Action Subsystem ==
  note: Change Log:
      | Oct 12, 2012  Created by Kevin Derry as a 1-input, 1-output block
      | Nov 30, 2012  dynamically configurable for 1 to 5 ports.
  note: Do not modify these blocks manually.  They
      | are generated programatically.  Changing the
      | number of blocks available or their names requires
      | corresponding changes to Callback and Initialization
      | routines.
      |
      | Do not change the "Display" tab of mask editor.  The
      | outport names are created programatically in the
      | "Initialize" section.
  In1 : Inport
  Action Port : ActionPort  ActionType=then
  In{2..5} (4 alike) : Ground
  Out{2..5} (4 alike) : Terminator
  Out1 : Outport
  wires:
  In1/1 -> Out1/1
  In2/1 -> Out2/1
  In3/1 -> Out3/1
  In4/1 -> Out4/1
  In5/1 -> Out5/1

== system DF002A_Swp/Swp/DF002A Sweep Function/ SwpPer1/Check GenHwTrq and VehSpd/If GenHwTrq=TRUE, Check Vehicle Speed Criteria/Switch Case Block/Start//Transition: Switch Case Action Subsystem /ScaleFactor Calculation/Then Action Subsystem ==
  note: Do not modify these blocks manually.  They
      | are generated programatically.  Changing the
      | number of blocks available or their names requires
      | corresponding changes to Callback and Initialization
      | routines.
      |
      | Do not change the "Display" tab of mask editor.  The
      | outport names are created programatically in the
      | "Initialize" section.
  note: Change Log:
      | Oct 12, 2012  Created by Kevin Derry as a 1-input, 1-output block
      | Nov 30, 2012  dynamically configurable for 1 to 5 ports.
  In1 : Inport
  Action Port : ActionPort  ActionType=else
  In{2..5} (4 alike) : Ground
  Out{2..5} (4 alike) : Terminator
  Out1 : Outport
  wires:
  In5/1 -> Out5/1
  In4/1 -> Out4/1
  In3/1 -> Out3/1
  In2/1 -> Out2/1
  In1/1 -> Out1/1

== system DF002A_Swp/Swp/DF002A Sweep Function/ SwpPer1/Check GenHwTrq and VehSpd/If GenHwTrq=TRUE, Check Vehicle Speed Criteria/Switch Case Block/Start//Transition: Switch Case Action Subsystem /if/CopyRight2 ==

== system DF002A_Swp/Swp/DF002A Sweep Function/ SwpPer1/Check GenHwTrq and VehSpd/If GenHwTrq=TRUE, Check Vehicle Speed Criteria/Switch Case Block/Start//Transition: Switch Case Action Subsystem /if/GetRefTmr100MicroSec32bit ==
  note: 1 count = 100 uSec
  note: seconds
  note: microseconds
  note: counts
  note: Wrap-to-zero
  note: GetRefTmr100MicroSec32bit
  Clock : Clock
  CopyRight2 : Subsystem  Description=|  mask(Copyright Information){none=on}
      | Copyright info block.                                               
      |                                                                     
      | Place copyright information at the top of every subsystem in design.
      mask prompts: none "No parameters"
      mask help: Place copyright information at the top of every subsystem in design.
      mask Display:
      | NxtrConf = 'Nexteer Confidential';
      | 
      | sys = bdroot; %handle for the current model ("system")
      | first = get_param(sys,'Created');
      | if(isempty(first))
      |     first = datestr(now,'yyyy');
      | else
      |     first = first(end-3:end);  %year is last four digits
      | end
      | 
      | last = get_param(sys,'LastModifiedDate');
      | if isempty(last)
      |     last = datestr(now,'yyyy');
      | else
      |     last = last(end-3:end);
      | end
      | 
      | if strcmp(first,last)
      |     fprintf('%s -- Copyright %s Nexteer',NxtrConf,first)
      | else
      |     fprintf('%s -- %s%s- %s Nexteer',NxtrConf,char(169),first,last)
      | end
  Count per uSec : Constant  Value=0.01
  Data Type Conversion1 : DataTypeConversion  OutDataTypeStr=uint32
  Divide1 : Product  Inputs=**
  Divide2 : Product  Inputs=*/
  Max Counts : Constant  Value=2^32-1
  Product1 : Product
  Product2 : Product
  Rounding : Rounding
  Subtract1 : Sum  Inputs=+-
  uSec per Sec : Constant  Value=1000000
  RefTmr : Outport
  wires:
  Product2/1 -> Subtract1/2
  Subtract1/1 -> Data Type Conversion1/1
  Rounding/1 -> Product2/1
  Divide2/1 -> Rounding/1
  Max Counts/1 -> Divide2/2, Product2/2
  Divide1/1 -> Divide2/1, Subtract1/1
  Product1/1 -> Divide1/1
  Clock/1 -> Product1/1
  Count per uSec/1 -> Divide1/2
  uSec per Sec/1 -> Product1/2
  Data Type Conversion1/1 -> RefTmr/1

== system DF002A_Swp/Swp/DF002A Sweep Function/ SwpPer1/Check GenHwTrq and VehSpd/If GenHwTrq=TRUE, Check Vehicle Speed Criteria/Switch Case Block/Dwell//Stop: Switch Case Action Subsystem1/If Action Subsystem/if/CopyRight2 ==

== system DF002A_Swp/Swp/DF002A Sweep Function/ SwpPer1/Check GenHwTrq and VehSpd/If GenHwTrq=TRUE, Check Vehicle Speed Criteria/Switch Case Block/Dwell//Stop: Switch Case Action Subsystem1/If Action Subsystem/if/GetRefTmr100MicroSec32bit ==
  note: 1 count = 100 uSec
  note: seconds
  note: microseconds
  note: counts
  note: Wrap-to-zero
  note: GetRefTmr100MicroSec32bit
  Clock : Clock
  CopyRight2 : Subsystem  Description=|  mask(Copyright Information){none=on}
      | Copyright info block.                                               
      |                                                                     
      | Place copyright information at the top of every subsystem in design.
      mask prompts: none "No parameters"
      mask help: Place copyright information at the top of every subsystem in design.
      mask Display:
      | NxtrConf = 'Nexteer Confidential';
      | 
      | sys = bdroot; %handle for the current model ("system")
      | first = get_param(sys,'Created');
      | if(isempty(first))
      |     first = datestr(now,'yyyy');
      | else
      |     first = first(end-3:end);  %year is last four digits
      | end
      | 
      | last = get_param(sys,'LastModifiedDate');
      | if isempty(last)
      |     last = datestr(now,'yyyy');
      | else
      |     last = last(end-3:end);
      | end
      | 
      | if strcmp(first,last)
      |     fprintf('%s -- Copyright %s Nexteer',NxtrConf,first)
      | else
      |     fprintf('%s -- %s%s- %s Nexteer',NxtrConf,char(169),first,last)
      | end
  Count per uSec : Constant  Value=0.01
  Data Type Conversion1 : DataTypeConversion  OutDataTypeStr=uint32
  Divide1 : Product  Inputs=**
  Divide2 : Product  Inputs=*/
  Max Counts : Constant  Value=2^32-1
  Product1 : Product
  Product2 : Product
  Rounding : Rounding
  Subtract1 : Sum  Inputs=+-
  uSec per Sec : Constant  Value=1000000
  RefTmr : Outport
  wires:
  Product2/1 -> Subtract1/2
  Subtract1/1 -> Data Type Conversion1/1
  Rounding/1 -> Product2/1
  Divide2/1 -> Rounding/1
  Max Counts/1 -> Divide2/2, Product2/2
  Divide1/1 -> Divide2/1, Subtract1/1
  Product1/1 -> Divide1/1
  Clock/1 -> Product1/1
  Count per uSec/1 -> Divide1/2
  uSec per Sec/1 -> Product1/2
  Data Type Conversion1/1 -> RefTmr/1

== system DF002A_Swp/Swp/DF002A Sweep Function/ SwpPer1/Check GenHwTrq and VehSpd/If GenHwTrq=TRUE, Check Vehicle Speed Criteria/Switch Case Block/Dwell//Stop: Switch Case Action Subsystem1/If Action Subsystem/if1/CopyRight2 ==

== system DF002A_Swp/Swp/DF002A Sweep Function/ SwpPer1/Check GenHwTrq and VehSpd/If GenHwTrq=TRUE, Check Vehicle Speed Criteria/Switch Case Block/Dwell//Stop: Switch Case Action Subsystem1/If Action Subsystem/if1/GetRefTmr100MicroSec32bit ==
  note: 1 count = 100 uSec
  note: seconds
  note: microseconds
  note: counts
  note: Wrap-to-zero
  note: GetRefTmr100MicroSec32bit
  Clock : Clock
  CopyRight2 : Subsystem  Description=|  mask(Copyright Information){none=on}
      | Copyright info block.                                               
      |                                                                     
      | Place copyright information at the top of every subsystem in design.
      mask prompts: none "No parameters"
      mask help: Place copyright information at the top of every subsystem in design.
      mask Display:
      | NxtrConf = 'Nexteer Confidential';
      | 
      | sys = bdroot; %handle for the current model ("system")
      | first = get_param(sys,'Created');
      | if(isempty(first))
      |     first = datestr(now,'yyyy');
      | else
      |     first = first(end-3:end);  %year is last four digits
      | end
      | 
      | last = get_param(sys,'LastModifiedDate');
      | if isempty(last)
      |     last = datestr(now,'yyyy');
      | else
      |     last = last(end-3:end);
      | end
      | 
      | if strcmp(first,last)
      |     fprintf('%s -- Copyright %s Nexteer',NxtrConf,first)
      | else
      |     fprintf('%s -- %s%s- %s Nexteer',NxtrConf,char(169),first,last)
      | end
  Count per uSec : Constant  Value=0.01
  Data Type Conversion1 : DataTypeConversion  OutDataTypeStr=uint32
  Divide1 : Product  Inputs=**
  Divide2 : Product  Inputs=*/
  Max Counts : Constant  Value=2^32-1
  Product1 : Product
  Product2 : Product
  Rounding : Rounding
  Subtract1 : Sum  Inputs=+-
  uSec per Sec : Constant  Value=1000000
  RefTmr : Outport
  wires:
  Product2/1 -> Subtract1/2
  Subtract1/1 -> Data Type Conversion1/1
  Rounding/1 -> Product2/1
  Divide2/1 -> Rounding/1
  Max Counts/1 -> Divide2/2, Product2/2
  Divide1/1 -> Divide2/1, Subtract1/1
  Product1/1 -> Divide1/1
  Clock/1 -> Product1/1
  Count per uSec/1 -> Divide1/2
  uSec per Sec/1 -> Product1/2
  Data Type Conversion1/1 -> RefTmr/1

== system DF002A_Swp/Swp/DF002A Sweep Function/ SwpPer1/Check GenHwTrq and VehSpd/If GenHwTrq=TRUE, Check Vehicle Speed Criteria/Switch Case Block/Start//Transition: Switch Case Action Subsystem /if/GetRefTmr100MicroSec32bit/CopyRight2 ==

== system DF002A_Swp/Swp/DF002A Sweep Function/ SwpPer1/Check GenHwTrq and VehSpd/If GenHwTrq=TRUE, Check Vehicle Speed Criteria/Switch Case Block/Dwell//Stop: Switch Case Action Subsystem1/If Action Subsystem/if/GetRefTmr100MicroSec32bit/CopyRight2 ==

== system DF002A_Swp/Swp/DF002A Sweep Function/ SwpPer1/Check GenHwTrq and VehSpd/If GenHwTrq=TRUE, Check Vehicle Speed Criteria/Switch Case Block/Dwell//Stop: Switch Case Action Subsystem1/If Action Subsystem/if1/GetRefTmr100MicroSec32bit/CopyRight2 ==
